simulink model "augmented_system"  (R2023a)
settings: Solver=VariableStepAuto  StartTime=0.0  StopTime=10.0  RelTol=1e-3
values from neighbouring files (symbols this model uses):
  a = [-1 6 ... (first row only)    [ex09.m]    (also in rankcheck_1.m = diag(eig(A)))
  b = [1; -3]    [ex09.m]
  c = [2 3]    [ex09.m]
  F = place(A,B,p)    [ex05.m]    (also in ex09.m = -R'*b'*P(1,1))
  G = gram(A,B)    [ex02.m]    (also in ex09.m = -R'*b'*P(1,2); ex11.m = subs(Gs))
  H1 = 0    [ex09.m]
settings Model: Creator=sebe  LastModifiedBy=vigro
settings DebuggingCC: UnconnectedInputMsg=warning  UnconnectedOutputMsg=warning  UnconnectedLineMsg=warning
settings ModelReferenceCC: EnableRefExpFcnMdlSchedulingChecks=on
settings RTWCC: DLArmComputeVersion=19.05

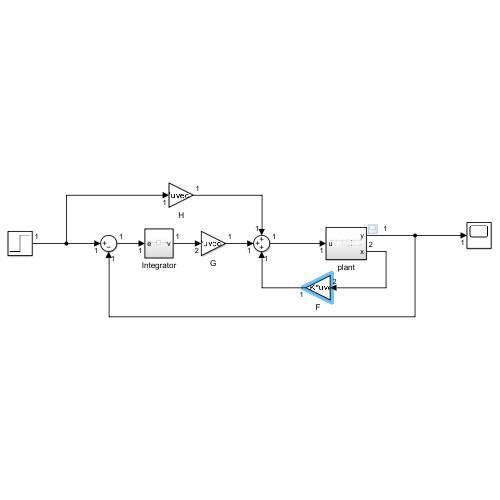
[thumbnail: Simulink's stored preview of the top-level diagram]
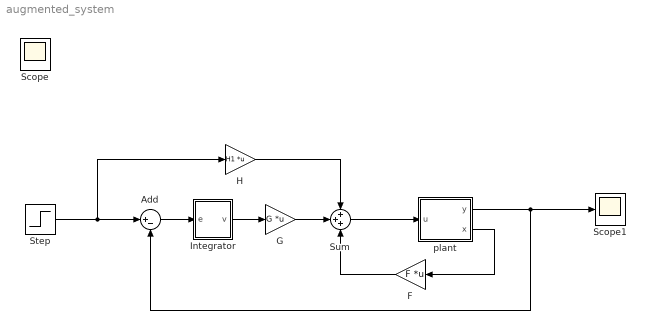
== system augmented_system ==
  Add : Sum  Inputs=|+-
  F : Gain  Gain=F  Multiplication=Matrix(K*u) (u vector)
  G : Gain  Gain=G  Multiplication=Matrix(K*u) (u vector)
  H : Gain  Gain=H1  Multiplication=Matrix(K*u) (u vector)
  Integrator : Subsystem
  Scope1 : Scope
  Step : Step  SampleTime=0
  Sum : Sum  Inputs=+++
  plant : Subsystem
  Scope : Scope
  wires:
  plant/1(y) -> Scope1/1, Add/2
  Sum/1 -> plant/1(u)
  Add/1 -> Integrator/1(e)
  Step/1 -> H/1, Add/1
  plant/2(x) -> F/1
  F/1 -> Sum/3
  Integrator/1(v) -> G/1
  G/1 -> Sum/2
  H/1 -> Sum/1

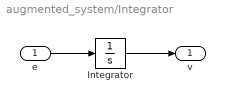
== system augmented_system/Integrator ==
  e : Inport
  Integrator : Integrator
  v : Outport
  wires:
  Integrator/1 -> v/1
  e/1 -> Integrator/1

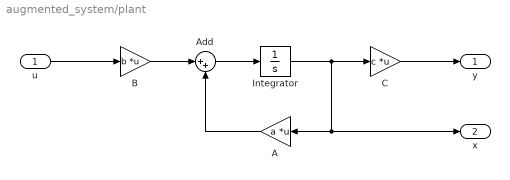
== system augmented_system/plant ==
  u : Inport
  A : Gain  Gain=a  Multiplication=Matrix(K*u) (u vector)
  Add : Sum  Inputs=|++
  B : Gain  Gain=b  Multiplication=Matrix(K*u) (u vector)
  C : Gain  Gain=c  Multiplication=Matrix(K*u) (u vector)
  Integrator : Integrator
  y : Outport
  x : Outport  Port=2
  wires:
  B/1 -> Add/1
  Add/1 -> Integrator/1
  A/1 -> Add/2
  u/1 -> B/1
  C/1 -> y/1
  Integrator/1 -> x/1, A/1, C/1
